simulink model "self_blancing_robot_simulink"  (R2020a)
settings: Solver=VariableStepAuto  StartTime=0.0  StopTime=100  RelTol=1e-3
values from neighbouring files (symbols this model uses):
  A = [0 1 0 0; A1 0 0 0; 0 0 0 1; -A2 0 0 0]    [simulation_variables.m]
  B = [0 -B1 0 B2]'    [simulation_variables.m]
  C = [1 0 0 0; 0 0 1 0]    [simulation_variables.m]
  K = lqr(A, B, Q, R)    [simulation_variables.m]
libraries: vrlib x15
settings Model: Creator=i  LastModifiedBy=i

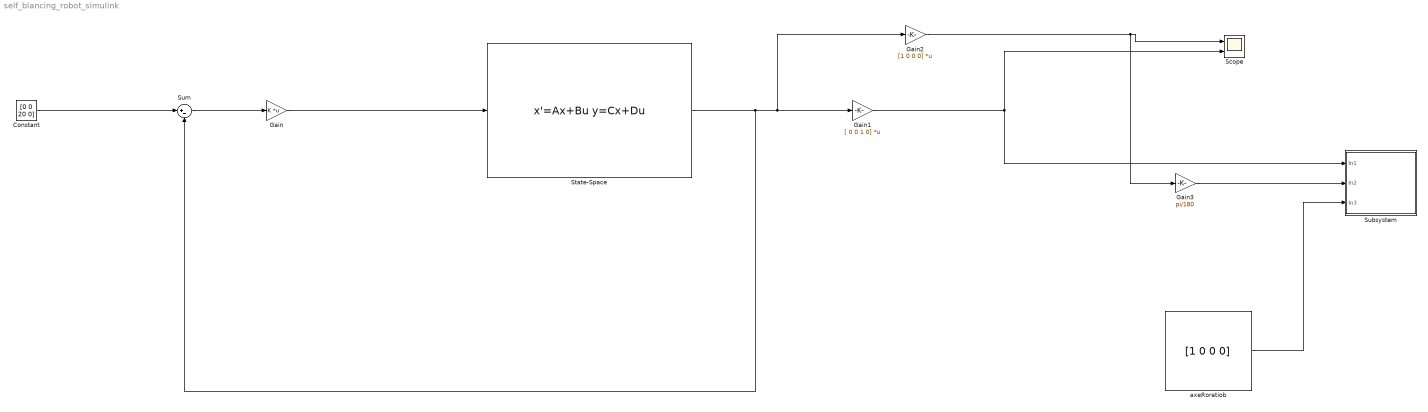
== system self_blancing_robot_simulink ==
  Constant : Constant  Value=[0 0 20 0]
  Gain : Gain  Gain=K  Multiplication=Matrix(K*u)
  Gain1 : Gain  Gain=[ 0 0 1 0]  Multiplication=Matrix(K*u)
  Gain2 : Gain  Gain=[1 0 0 0]  Multiplication=Matrix(K*u)
  Gain3 : Gain  Gain=pi/180
  Scope : Scope  NumInputPorts=2
  State-Space : StateSpace  A=A  B=B  C=eye(4)  D=[0 0 0 0]'  InitialCondition=[20 0 0 0]
  Subsystem : Subsystem
  Sum : Sum  Inputs=|+-
  axeRoratiob : Constant  Value=[1 0 0 0]  VectorParams1D=off  OutDataTypeStr=Inherit: Inherit via back propagation
  wires:
  axeRoratiob/1 -> Subsystem/3(In3)
  State-Space/1 -> Sum/2, Gain2/1, Gain1/1
  Constant/1 -> Sum/1
  Sum/1 -> Gain/1
  Gain/1 -> State-Space/1
  Gain2/1 -> Gain3/1, Scope/1
  Gain1/1 -> Subsystem/1(In1), Scope/2
  Gain3/1 -> Subsystem/2(In2)

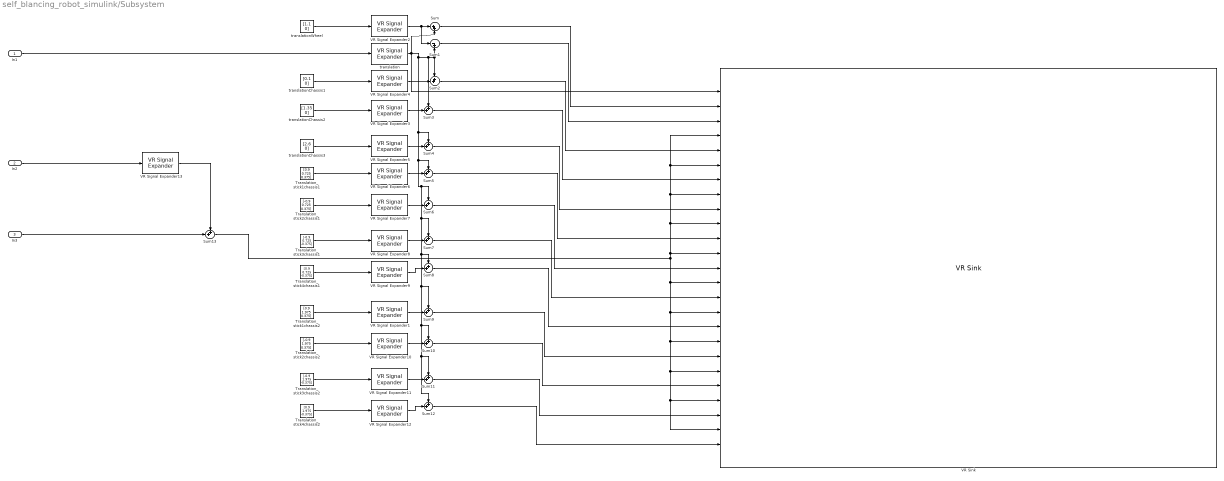
== system self_blancing_robot_simulink/Subsystem ==
  In1 : Inport
  In2 : Inport  Port=2
  In3 : Inport  Port=3
  Sum : Sum  Inputs=|++
  Sum1 : Sum  Inputs=|-+
  Sum{2..13} (12 alike) : Sum  Inputs=++|
  Translation_stick1chassis1 : Constant  Value=[0.9 0.725 0.375]  OutDataTypeStr=Inherit: Inherit via back propagation
  Translation_stick1chassis2 : Constant  Value=[0.9 1.975 0.375]  OutDataTypeStr=Inherit: Inherit via back propagation
  Translation_stick2chassis1 : Constant  Value=[-0.9 0.725 0.375]  OutDataTypeStr=Inherit: Inherit via back propagation
  Translation_stick2chassis2 : Constant  Value=[-0.9 1.975 0.375]  OutDataTypeStr=Inherit: Inherit via back propagation
  Translation_stick3chassis1 : Constant  Value=[-0.9 0.725 -0.375]  OutDataTypeStr=Inherit: Inherit via back propagation
  Translation_stick3chassis2 : Constant  Value=[-0.9 1.975 -0.375]  OutDataTypeStr=Inherit: Inherit via back propagation
  Translation_stick4chassis1 : Constant  Value=[0.9 0.725 -0.375]  OutDataTypeStr=Inherit: Inherit via back propagation
  Translation_stick4chassis2 : Constant  Value=[0.9 1.975 -0.375]  OutDataTypeStr=Inherit: Inherit via back propagation
  VR Signal Expander{1,6..12} (8 alike) : vrlib/VR Signal Expander  outwidth=3  outidx=[1 2 3]
  VR Signal Expander13 : vrlib/VR Signal Expander  outwidth=4  outidx=[4]
  VR Signal Expander{2..5} (4 alike) : vrlib/VR Signal Expander  outwidth=3  outidx=[1 3]
  VR Sink : vrlib/VR Sink  InstantiateOnLoad=on  SampleTime=0.01  ViewEnable=on  RemoteChange=off  RemoteView=off  FieldsWritten=stick_wheels.translation.3.1.1.double#R_wheel.translation.3.1.1.double#L_wheel.translation.3.1.1.double#chassis1.rotation.4.1.1.double#chassis1.translation.3.1.1.double#chassis2.rotation.4.1.1.double#chassis2.translation.3.1.1.double#chassis3.rotation.4.1.1.double#chassis3.translation.3.1.1.double#stick1_chassis1.rotation.4.1.1.double#stick1_chassis1.translation.3.1.1.double#stick2_chassis1.rotation.4.1.1.double#stick2_chassis1.translation.3.1.1.double#stick3_chassis1.rotation.4.1.1.double#stick3_chassis1.translation.3.1.1.double#stick4_chassis1.rotation.4.1.1.double#stick4_chassis1.translation.3.1.1.double#stick1_chassis2.rotation.4.1.1.double#stick1_chassis2.translation.3.1.1.double#stick2_chassis2.rotation.4.1.1.double#stick2_chassis2.translation.3.1.1.double#stick3_chassis2.rotation.4.1.1.double#stick3_chassis2.translation.3.1.1.double#stick4_chassis2.rotation.4.1.1.double#stick4_chassis2.translation.3.1.1.double  WorldFileName=C:\Users\i\Desktop\selfBalancingrobot\self_blancing_robot_VRLM.wrl  AutoView=off  VideoDimensions=[]  AllowVariableSize=off  FigureProperties="{'Position', 'Name', 'Viewpoint', 'CameraBound', 'CameraDirection', 'CameraPosition', 'CameraUpVector', 'ZoomFactor', 'Antialiasing', 'Headlight', 'Lighting', 'NavPanel', 'Sound', 'StatusBar', 'Stereo3D', 'Stereo3DCameraOffset', 'Stereo3DHIT', 'ToolBar', 'Textures', 'Transparency', 'Triad', 'Wireframe', 'NavZones', 'NavMode', 'NavSpeed', 'CaptureFileFormat', 'CaptureFileName', 'Record2DCompressMethod', 'Record2DCompressQuality', 'Record2D', 'Record2DFileName', 'Record2DFPS'; [1.0000000000000000e+00   7.1666666666666742e+01   1.2800000000000000e+03   5.5733333333333326e+02], '', '', 'on', [2.1026147350291613e-01  -9.2143805185104875e-04  -9.7764475332932699e-01], [-1.0186571028085920e+01   1.3714321519054677e+00   3.8484852733865743e+01], [1.4520545660521700e-01   9.8893753943601104e-01   3.0297169279400266e-02], [1.0000000000000000e+00], 'on', 'on', 'on', 'halfbar', 'on', 'on', 'off', [1.0000000149011612e-01], [0.0000000000000000e+00], 'on', 'on', 'on', 'none', 'off', 'off', 'fly', 'normal', 'tif', '%f_anim_%n.tif', 'auto', [7.5000000000000000e+01], 'off', '%f_anim_%n.avi', 'auto'}"
  translation : vrlib/VR Signal Expander  outwidth=3  outidx=[3]
  translationChassis1 : Constant  Value=[0.1 0]  OutDataTypeStr=Inherit: Inherit via back propagation
  translationChassis2 : Constant  Value=[1.35 0]  OutDataTypeStr=Inherit: Inherit via back propagation
  translationChassis3 : Constant  Value=[2.6 0]  OutDataTypeStr=Inherit: Inherit via back propagation
  translationWheel : Constant  Value=[1.1 0]  OutDataTypeStr=Inherit: Inherit via back propagation
  wires:
  Translation_stick2chassis2/1 -> VR Signal Expander10/1
  translationWheel/1 -> VR Signal Expander2/1
  Sum13/1 -> VR Sink/24, VR Sink/22, VR Sink/20, VR Sink/18, VR Sink/16, VR Sink/14, VR Sink/10, VR Sink/8, VR Sink/4, VR Sink/6, VR Sink/12
  Translation_stick4chassis1/1 -> VR Signal Expander9/1
  VR Signal Expander8/1 -> Sum7/2
  translation/1 -> Sum/2, VR Sink/1, Sum9/1, Sum10/1, Sum12/1, Sum11/1, Sum8/1, Sum7/1, Sum6/1, Sum5/1, Sum4/1, Sum3/1, Sum2/1, Sum1/2
  VR Signal Expander5/1 -> Sum4/2
  Translation_stick1chassis1/1 -> VR Signal Expander6/1
  VR Signal Expander3/1 -> Sum3/2
  Sum2/1 -> VR Sink/5
  Sum1/1 -> VR Sink/3
  VR Signal Expander4/1 -> Sum2/2
  VR Signal Expander6/1 -> Sum5/2
  VR Signal Expander10/1 -> Sum10/2
  translationChassis1/1 -> VR Signal Expander4/1
  VR Signal Expander2/1 -> Sum1/1, Sum/1
  Translation_stick1chassis2/1 -> VR Signal Expander1/1
  translationChassis2/1 -> VR Signal Expander3/1
  translationChassis3/1 -> VR Signal Expander5/1
  Sum5/1 -> VR Sink/11
  In1/1 -> translation/1
  VR Signal Expander7/1 -> Sum6/2
  VR Signal Expander9/1 -> Sum8/2
  Sum3/1 -> VR Sink/7
  VR Signal Expander11/1 -> Sum11/2
  Sum7/1 -> VR Sink/15
  Translation_stick2chassis1/1 -> VR Signal Expander7/1
  Translation_stick3chassis2/1 -> VR Signal Expander11/1
  VR Signal Expander13/1 -> Sum13/1
  Sum8/1 -> VR Sink/17
  VR Signal Expander12/1 -> Sum12/2
  Sum6/1 -> VR Sink/13
  Translation_stick3chassis1/1 -> VR Signal Expander8/1
  Sum4/1 -> VR Sink/9
  Sum9/1 -> VR Sink/19
  VR Signal Expander1/1 -> Sum9/2
  Sum/1 -> VR Sink/2
  Sum11/1 -> VR Sink/23
  Sum10/1 -> VR Sink/21
  Translation_stick4chassis2/1 -> VR Signal Expander12/1
  Sum12/1 -> VR Sink/25
  In2/1 -> VR Signal Expander13/1
  In3/1 -> Sum13/2
